simulink model "state_observer_without_feedback"  (R2019a)
settings: Solver=ode45  StartTime=0.0  StopTime=100  RelTol=1e-3  EnableMultiTasking=on
undefined symbols (not defined in the file or in its folder): a, b, c, l
libraries: simulink x2
settings Model: Creator=Lazaros  LastModifiedBy=rohit
settings DataIOCC: LimitDataPoints=on  SaveFormat=Array  ReturnWorkspaceOutputs=off
settings OptimizationCC: LifeSpan=inf
settings DebuggingCC: UnderspecifiedInitializationDetection=Classic  MergeDetectMultiDrivingBlocksExec=none  SolverPrmCheckMsg=warning  StateNameClashWarn=warning  SFUnexpectedBacktrackingDiag=warning  SFNoUnconditionalDefaultTransitionDiag=warning  SFExecutionAtInitializationDiag=none  ArithmeticOperatorsInVariantConditions=warning
settings HardwareCC: ProdBitPerPointer=32  ProdBitPerSizeT=32  ProdBitPerPtrDiffT=32  ProdLargestAtomicFloat=None  ProdIntDivRoundTo=Undefined  ProdEndianess=Unspecified  ProdWordSize=32  ProdHWDeviceType=32-bit Generic
settings ModelReferenceCC: PropagateSignalLabelsOutOfModel=off
settings SFSimCC: SimUseLocalCustomCode=off
settings RTWCC: RTWUseLocalCustomCode=off
settings CodeAppCC: StateflowObjectComments=on
settings GRTTargetCC: TargetLangStandard=C89/C90 (ANSI)  GeneratePreprocessorConditionals=Disable all
settings ConfigComp: CovMetricSettings=dw  CovHtmlReporting=on  CovSaveCumulativeToWorkspaceVar=on  CovSaveSingleToWorkspaceVar=on  CovExternalEMLEnable=off

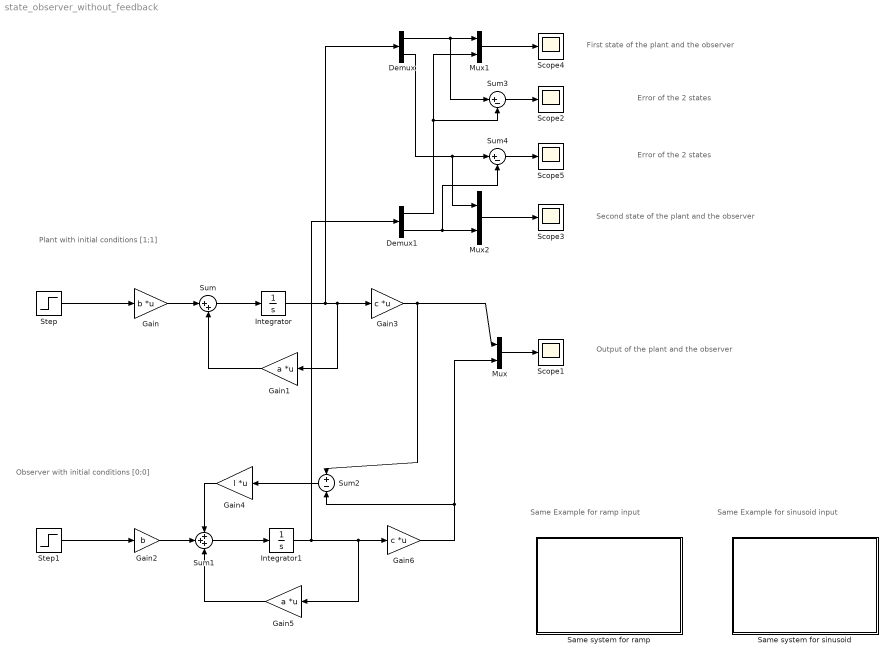
== system state_observer_without_feedback ==
  note: First state of the plant and the observer
  note: Output of the plant and the observer
  note: Second state of the plant and the observer
  note: Error of the 2 states
  note: Observer with initial conditions
      | [0;0]
  note: Plant with initial conditions
      | [1;1]
  note: Error of the 2 states
  note: Same Example for ramp input
  note: Same Example for sinusoid input
  Demux : Demux  Outputs=2
  Demux1 : Demux  Outputs=2
  Gain : Gain  Gain=b  Multiplication=Matrix(K*u)
  Gain1 : Gain  Gain=a  Multiplication=Matrix(K*u)
  Gain2 : Gain  Gain=b
  Gain3 : Gain  Gain=c  Multiplication=Matrix(K*u)
  Gain4 : Gain  Gain=l  Multiplication=Matrix(K*u)
  Gain5 : Gain  Gain=a  Multiplication=Matrix(K*u)
  Gain6 : Gain  Gain=c  Multiplication=Matrix(K*u)
  Integrator : Integrator  InitialCondition=[1;1]
  Integrator1 : Integrator
  Mux : Mux  Inputs=2
  Mux1 : Mux  Inputs=2
  Mux2 : Mux  Inputs=2
  Same system for ramp : Subsystem
      mask Display: image('obs.png')
  Same system for sinusoid : Subsystem
      mask Display: image('obs.png')
  Scope{1..5} (5 alike) : Scope
  Step : Step  Time=0  SampleTime=0
  Step1 : Step  Time=0  SampleTime=0
  Sum : Sum  Inputs=|++
  Sum1 : Sum  Inputs=+++
  Sum2 : Sum  Inputs=+-
  Sum3 : Sum  Inputs=|+-
  Sum4 : Sum  Inputs=|+-
  wires:
  Step/1 -> Gain/1
  Gain/1 -> Sum/1
  Sum/1 -> Integrator/1
  Integrator/1 -> Demux/1, Gain1/1, Gain3/1
  Gain1/1 -> Sum/2
  Step1/1 -> Gain2/1
  Sum1/1 -> Integrator1/1
  Gain2/1 -> Sum1/2
  Gain3/1 -> Sum2/1, Mux/1
  Sum2/1 -> Gain4/1
  Gain4/1 -> Sum1/1
  Integrator1/1 -> Demux1/1, Gain6/1, Gain5/1
  Gain5/1 -> Sum1/3
  Gain6/1 -> Mux/2, Sum2/2
  Sum3/1 -> Scope2/1
  Mux/1 -> Scope1/1
  Demux/1 -> Sum3/1, Mux1/1
  Demux1/1 -> Mux1/2, Sum3/2
  Mux1/1 -> Scope4/1
  Demux/2 -> Mux2/1, Sum4/1
  Demux1/2 -> Mux2/2, Sum4/2
  Mux2/1 -> Scope3/1
  Sum4/1 -> Scope5/1

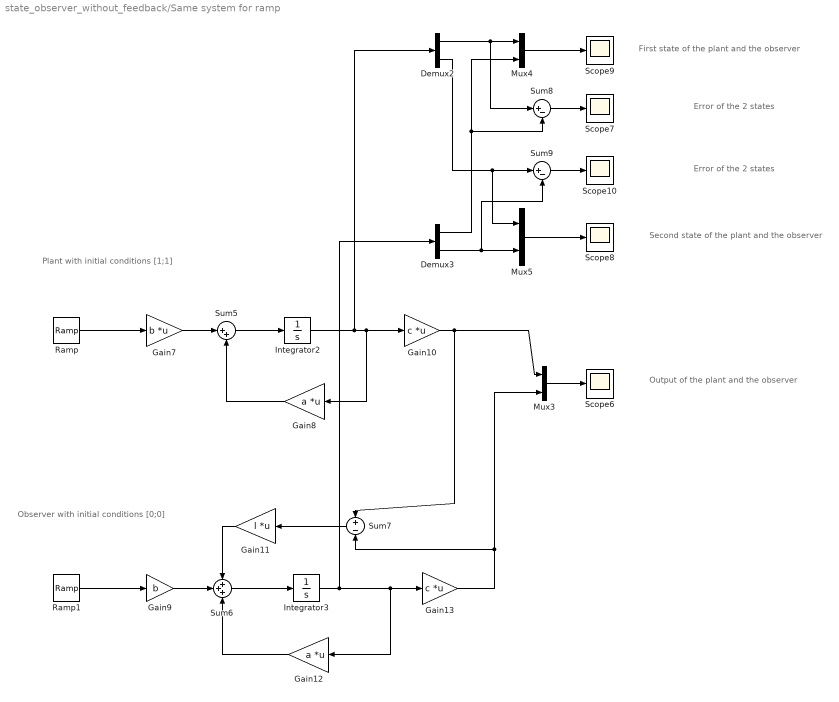
== system state_observer_without_feedback/Same system for ramp ==
  note: First state of the plant and the observer
  note: Output of the plant and the observer
  note: Second state of the plant and the observer
  note: Error of the 2 states
  note: Observer with initial conditions
      | [0;0]
  note: Plant with initial conditions
      | [1;1]
  note: Error of the 2 states
  Demux2 : Demux  Outputs=2
  Demux3 : Demux  Outputs=2
  Gain10 : Gain  Gain=c  Multiplication=Matrix(K*u)
  Gain11 : Gain  Gain=l  Multiplication=Matrix(K*u)
  Gain12 : Gain  Gain=a  Multiplication=Matrix(K*u)
  Gain13 : Gain  Gain=c  Multiplication=Matrix(K*u)
  Gain7 : Gain  Gain=b  Multiplication=Matrix(K*u)
  Gain8 : Gain  Gain=a  Multiplication=Matrix(K*u)
  Gain9 : Gain  Gain=b
  Integrator2 : Integrator  InitialCondition=[1;1]
  Integrator3 : Integrator
  Mux3 : Mux  Inputs=2
  Mux4 : Mux  Inputs=2
  Mux5 : Mux  Inputs=2
  Ramp : simulink/Sources/Ramp  slope=1  start=0  InitialOutput=0
  Ramp1 : simulink/Sources/Ramp  slope=1  start=0  InitialOutput=0
  Scope{6..10} (5 alike) : Scope
  Sum5 : Sum  Inputs=|++
  Sum6 : Sum  Inputs=+++
  Sum7 : Sum  Inputs=+-
  Sum8 : Sum  Inputs=|+-
  Sum9 : Sum  Inputs=|+-
  wires:
  Ramp/1 -> Gain7/1
  Gain7/1 -> Sum5/1
  Sum5/1 -> Integrator2/1
  Integrator2/1 -> Demux2/1, Gain8/1, Gain10/1
  Gain8/1 -> Sum5/2
  Ramp1/1 -> Gain9/1
  Sum6/1 -> Integrator3/1
  Gain9/1 -> Sum6/2
  Gain10/1 -> Sum7/1, Mux3/1
  Sum7/1 -> Gain11/1
  Gain11/1 -> Sum6/1
  Integrator3/1 -> Demux3/1, Gain13/1, Gain12/1
  Gain12/1 -> Sum6/3
  Sum9/1 -> Scope10/1
  Demux3/1 -> Mux4/2, Sum8/2
  Demux2/2 -> Mux5/1, Sum9/1
  Demux3/2 -> Mux5/2, Sum9/2
  Gain13/1 -> Mux3/2, Sum7/2
  Mux3/1 -> Scope6/1
  Mux5/1 -> Scope8/1
  Mux4/1 -> Scope9/1
  Sum8/1 -> Scope7/1
  Demux2/1 -> Sum8/1, Mux4/1

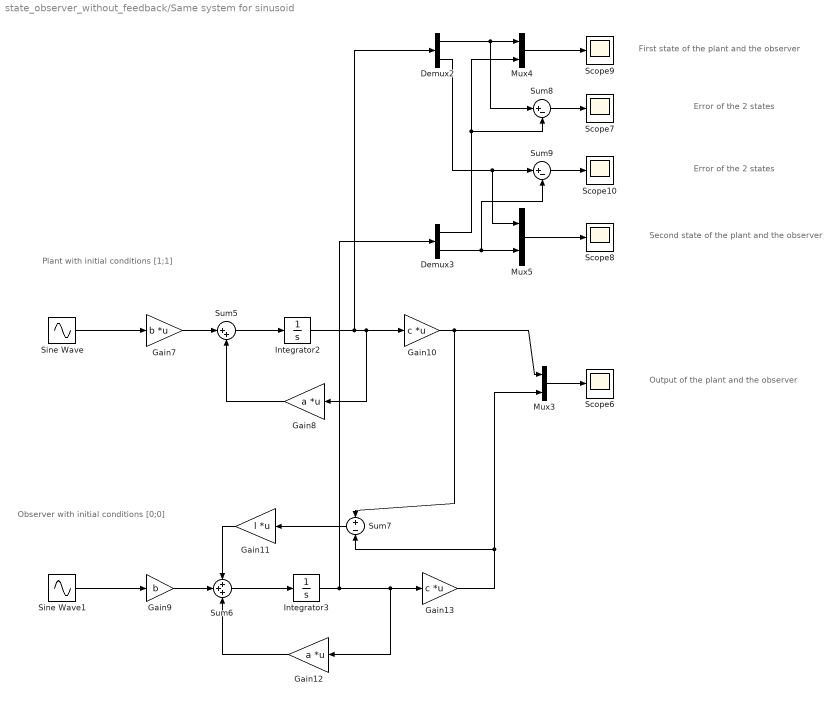
== system state_observer_without_feedback/Same system for sinusoid ==
  note: First state of the plant and the observer
  note: Output of the plant and the observer
  note: Second state of the plant and the observer
  note: Error of the 2 states
  note: Observer with initial conditions
      | [0;0]
  note: Plant with initial conditions
      | [1;1]
  note: Error of the 2 states
  Demux2 : Demux  Outputs=2
  Demux3 : Demux  Outputs=2
  Gain10 : Gain  Gain=c  Multiplication=Matrix(K*u)
  Gain11 : Gain  Gain=l  Multiplication=Matrix(K*u)
  Gain12 : Gain  Gain=a  Multiplication=Matrix(K*u)
  Gain13 : Gain  Gain=c  Multiplication=Matrix(K*u)
  Gain7 : Gain  Gain=b  Multiplication=Matrix(K*u)
  Gain8 : Gain  Gain=a  Multiplication=Matrix(K*u)
  Gain9 : Gain  Gain=b
  Integrator2 : Integrator  InitialCondition=[1;1]
  Integrator3 : Integrator
  Mux3 : Mux  Inputs=2
  Mux4 : Mux  Inputs=2
  Mux5 : Mux  Inputs=2
  Scope{6..10} (5 alike) : Scope
  Sine Wave : Sin  Amplitude=3  SampleTime=0
  Sine Wave1 : Sin  Amplitude=3  SampleTime=0
  Sum5 : Sum  Inputs=|++
  Sum6 : Sum  Inputs=+++
  Sum7 : Sum  Inputs=+-
  Sum8 : Sum  Inputs=|+-
  Sum9 : Sum  Inputs=|+-
  wires:
  Sine Wave/1 -> Gain7/1
  Gain7/1 -> Sum5/1
  Sum5/1 -> Integrator2/1
  Integrator2/1 -> Demux2/1, Gain8/1, Gain10/1
  Gain8/1 -> Sum5/2
  Sum6/1 -> Integrator3/1
  Gain9/1 -> Sum6/2
  Gain10/1 -> Sum7/1, Mux3/1
  Sum7/1 -> Gain11/1
  Gain11/1 -> Sum6/1
  Integrator3/1 -> Demux3/1, Gain13/1, Gain12/1
  Gain12/1 -> Sum6/3
  Sum9/1 -> Scope10/1
  Demux3/1 -> Mux4/2, Sum8/2
  Demux2/2 -> Mux5/1, Sum9/1
  Demux3/2 -> Mux5/2, Sum9/2
  Gain13/1 -> Mux3/2, Sum7/2
  Mux3/1 -> Scope6/1
  Mux5/1 -> Scope8/1
  Mux4/1 -> Scope9/1
  Sum8/1 -> Scope7/1
  Demux2/1 -> Sum8/1, Mux4/1
  Sine Wave1/1 -> Gain9/1
